simulink model "SimulinkProjectQ6"  (R2023a)
settings: Solver=VariableStepAuto  StartTime=0.0  StopTime=10.0  RelTol=1e-3
settings Model: Creator=phile  LastModifiedBy=phile

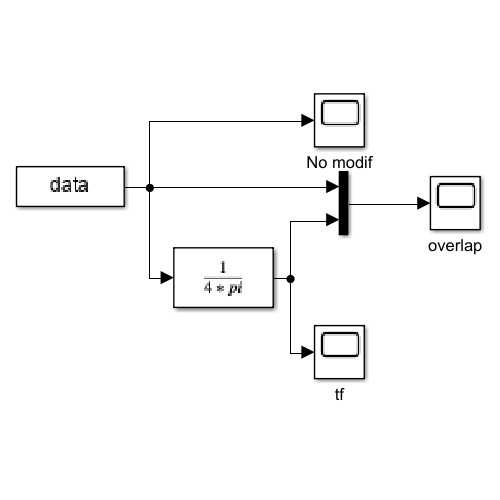
[thumbnail: Simulink's stored preview of the top-level diagram]
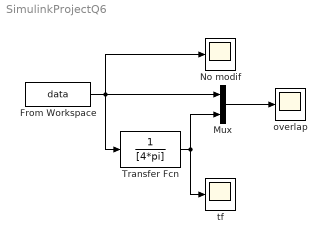
== system SimulinkProjectQ6 ==
  From Workspace : FromWorkspace  VariableName=data  SampleTime=0.001
  Mux : Mux  Inputs=2
  No modif : Scope
  Transfer Fcn : TransferFcn  Denominator=[4*pi]
  overlap : Scope
  tf : Scope
  wires:
  From Workspace/1 -> Mux/1, Transfer Fcn/1, No modif/1
  Transfer Fcn/1 -> tf/1, Mux/2
  Mux/1 -> overlap/1
